simulink model "TRN_V3"  (R2022a)
settings: Solver=FixedStepAuto  StartTime=0.0  StopTime=300  FixedStep=0.04  RelTol=1e-3
PreLoadFcn:
  | load('BusStructureTRNsensor.mat')
InitFcn:
  | %load TRNDataBusPILS.mat
  | %addpath(genpath(cd))
  | 
  | % Add DataBus Path
  | addpath(',,/');
  | addpath('../MAP/');
  | addpath('../MAP/MAP_DB');
  | addpath('../MAP/DVOF');
  | addpath(genpath(cd));
  | load('BusStructureTRN.mat');
  | load('BusStructureDatapump.mat');
undefined symbols (not defined in the file or in its folder): Altitude_INS, INSDataNotValid, Latitude_INS, Longitude_INS, RALTValid, TRN, TRNlib
libraries: simulink_extras x38, aerolibconvert2 x20, dspstat3 x3, sharedtransform x2
(part 3 of 3)

== stateflow chart TRN_V3/TRN/TRNSchedulerDTNS1 ==
  state Operation_In_Flight
    state Check_On_Terrain_Map [parallel]
      en, du:  Out_TRNOutput.AircraftOffTerrainMap = CheckOffTerrainMap(In_TRNInput.Latitude_INS, In_TRNInput.Longitude_INS);
      settings: executionOrder=1
    state Terrain_Referenced_Navigation [parallel]
      settings: executionOrder=2
      state On_Terrain_Map
        state AcquisitionCSU
          state Batch_On
            state CollectProfile [parallel]
              en, du: [Out_TRNDatapump.MAD, Out_TRNDatapump.profileCnt, posUpdate, Out_TRNDatapump.residual] =...
              AcquisitionCSU(In_TRNInput,In_TRNDatapump)
              settings: executionOrder=1
            state CorrelationAnalysis [parallel]
              settings: executionOrder=2
              state BatchUpdate_On
                en, du: Out_TRNOutput.TRNEstOfINSLatitudeErr = -posUpdate(1) * 180/pi;
                Out_TRNOutput.TRNEstOfINSLongitudeErr = -posUpdate(2) * 180/pi;
                Out_TRNDatapump.profileCnt = 0;
                Out_TRNOutput.NavigationMode = false;
                Out_TRNOutput.AircraftPositionCorrectionValid = true;
                Out_Pmatrix = InitPmatrix();
              state BatchUpdate_Off
                en, du: Out_TRNOutput.TRNEstOfINSLatitudeErr = 0.0;
                Out_TRNOutput.TRNEstOfINSLongitudeErr = 0.0;
                Out_TRNOutput.NavigationMode = true;
                Out_TRNOutput.AircraftPositionCorrectionValid = false;
                Out_Pmatrix = InitPmatrix();
              (default) -> (junction 198)
              (junction 198) -> BatchUpdate_On [order 1] : [(Out_TRNDatapump.MAD <= 50&&...
                  | Out_TRNDatapump.profileCnt >= 20) || ...
                  |  (In_TRNInput.GPSDataNotValid == 0 && ...
                  | Out_TRNDatapump.MAD <= 50&&...
                  | Out_TRNDatapump.profileCnt >= 5)]
              (junction 198) -> BatchUpdate_Off [order 2]
          state Batch_Idle
            entry: Out_TRNOutput.TRNEstOfINSLatitudeErr = 0.0;
            Out_TRNOutput.TRNEstOfINSLongitudeErr = 0.0;
            Out_TRNOutput.NavigationMode = true;
            Out_TRNOutput.AircraftPositionCorrectionValid = false;
          (default) -> Batch_On
          Batch_Idle -> Batch_On : after(24, tick)
          Batch_On -> Batch_Idle : after(1, tick)
        state TrackingCSU
          state ContinuousUpdate [parallel]
            en,du:  [xu,Pmatrix,residual,latINSErrTRN,lonINSErrTRN, ...
            altINSErrTRN,hUncertainty,vUncertainty, Out_TRNDatapump.TimeTag_Prev, Out_TRNDatapump.Result_Prev] = ...
            TrackingCSU(In_TRNInput,In_Pmatrix,Qmatrix,Rmatrix, In_TRNDatapump);
            [continuousValid, Out_TRNOutput.NavigationMode]...
            = CheckValidity( hUncertainty, In_TRNInput.INSDataNotValid);
            settings: executionOrder=1
          state ValidityCheck [parallel]
            settings: executionOrder=2
            state ContinuousValid
              en, du:
              Out_TRNOutput.TRNEstOfINSLatitudeErr = latINSErrTRN * 180/pi;
              Out_TRNOutput.TRNEstOfINSLongitudeErr = lonINSErrTRN * 180/pi;
              Out_TRNOutput.TRNEstOfINSAltitudeErr = altINSErrTRN;
              Out_TRNOutput.AircraftPositionCorrectionValid = true;
            state ContinuousInValid
              en, du:
              Out_TRNOutput.TRNEstOfINSLatitudeErr = 0.0;
              Out_TRNOutput.TRNEstOfINSLongitudeErr = 0.0;
              Out_TRNOutput.TRNEstOfINSAltitudeErr = 0.0;
              Out_TRNOutput.AircraftPositionCorrectionValid = false;
            (default) -> ContinuousValid
            ContinuousValid -> ContinuousInValid : [continuousValid == false]
            ContinuousInValid -> ContinuousValid : [continuousValid == true]
          state UpdateContinuousParam [parallel]
            en, du:
            Out_TRNOutput.TRNHorUncertainty = hUncertainty * 6378000 * 25;
            Out_TRNOutput.TRNVerticalUncertainty = vUncertainty * 25;
            Out_TRNDatapump.xu = xu;
            Out_TRNDatapump.residual = residual;
            Out_Pmatrix = Pmatrix;
            %Out_TRNOutput.TRN_valid = TRN_valid;
            settings: executionOrder=3
        (default) -> AcquisitionCSU
        TrackingCSU -> AcquisitionCSU : [In_TRNOutput.NavigationMode == true]
        AcquisitionCSU -> TrackingCSU : [In_TRNOutput.NavigationMode == false]
      state Of_fTerrain_Map
      (default) -> On_Terrain_Map
      On_Terrain_Map -> Of_fTerrain_Map : [Out_TRNOutput.AircraftOffTerrainMap == true]
      Of_fTerrain_Map -> On_Terrain_Map : [Out_TRNOutput.AircraftOffTerrainMap == false]
  state Flight_Idle
    en, du:
    Out_TRNOutput.AircraftOffTerrainMap = CheckOffTerrainMap(In_TRNInput.Latitude_INS, In_TRNInput.Longitude_INS);
    Out_TRNOutput.TRN_valid = true;
    Out_TRNOutput.TRNEstOfINSLatitudeErr = 0.0;
    Out_TRNOutput.TRNEstOfINSLongitudeErr = 0.0;
    Out_TRNOutput.TRNEstOfINSAltitudeErr = 0.0;
    Out_TRNOutput.NavigationMode = false;
    Out_TRNOutput.AircraftPositionCorrectionValid = false;
  state [xu,Out_Pmatrix,residual,latINSErrTRN,lonINSErrTRN,altINSErrTRN,hUncertainty,vUncertainty,TimeTag_Prev,Result_Prev] = TrackingCSU(In_TRNInput,In_Pmatrix,Qmatrix,Rmatrix,In_TRNDatapump) [function]
  state [MAD,profileCnt,posUpdate,residual] = AcquisitionCSU(In_TRNInput,In_TRNDatapump) [function]
  (default) -> Operation_In_Flight
  Operation_In_Flight -> Flight_Idle : [In_TRNInput.WeightOnWheels == 1]
  Flight_Idle -> Operation_In_Flight : [In_TRNInput.WeightOnWheels == 0]
  data: In_TRNInput function_input Bus: TRNInput size=1 =0; In_Pmatrix function_input double size=[15 15]; Qmatrix function_input double size=[6 6]; Rmatrix function_input double size=1; xu function_output; Out_Pmatrix function_output; residual function_output; latINSErrTRN function_output; lonINSErrTRN function_output; altINSErrTRN function_output; hUncertainty function_output; vUncertainty function_output; In_TRNDatapump function_input Bus: TRNDatapump size=1; TimeTag_Prev function_output; Result_Prev function_output; In_TRNInput function_input Bus: TRNInput size=1 =0; In_TRNDatapump function_input Bus: TRNDatapump size=1 =0; MAD function_output; profileCnt function_output; posUpdate function_output; residual function_output; hUncertaintyTRN function_input; INSDataNotValid function_input; valid function_output; navigationMode function_output; Pmat function_output double size=[15 15]; lat function_input; lon function_input; AircraftOffTerrainMap function_output; In_TRNInput input Bus: TRNInput; In_TRNOutput input Bus: TRNOutput; In_TRNDatapump input Bus: TRNDatapump; In_Pmatrix input double size=[15 15]; Out_TRNOutput output Bus: TRNOutput; Out_TRNDatapump output Bus: TRNDatapump; Qmatrix input double size=[6 6]; Rmatrix input double size=1; vUncertainty local double; lonINSErrTRN local double; latINSErrTRN local double; hUncertainty local double; altINSErrTRN local double; posUpdate local double; continuousValid local boolean; residual local double; xu local double size=15; Pmatrix local double size=[15 15]; Out_Pmatrix output double size=[15 15]
  function [valid, navigationMode] = CheckValidity(hUncertaintyTRN, INSDataNotValid):
    | % function [valid, navigationMode] = CheckValidity(hUncertaintyTRN, vUncertaintyTRN, residualTRN)
    | 
    | % persistent invalidCnt
    | % if(isempty(invalidCnt))
    | %     invalidCnt = 0;
    | % end
    | % 
    | % weightedResidual = abs(residualTRN)/vUncertaintyTRN;
    | % 
    | % if(vUncertainty > 1 && weightedResidual > 35)
    | %     valid = false;
    | %     invalidCnt = invalidCnt + 1;
    | % else
    | %     valid = true;
    | %     invalidCnt = 0;
    | % end
    | % 
    | % if (invalidCnt >= 50)
    | %     navigationMode = true;
    | % else
    | %     navigationMode = false;
    | % end
    | % 
    | % end
    | 
    | function [valid, navigationMode] = CheckValidity(hUncertaintyTRN, INSDataNotValid)
    | 
    | persistent invalidCnt
    | if(isempty(invalidCnt))
    |     invalidCnt = 0;
    | end
    | 
    | if(hUncertaintyTRN > (256 * 6378000 * 25)) || INSDataNotValid == 1
    | % if(hUncertaintyTRN > (256))
    |     valid = false;
    |     invalidCnt = invalidCnt + 1;
    | else
    |     valid = true;
    |     invalidCnt = 0;
    | end
    | 
    | if (invalidCnt >= 50) || INSDataNotValid == 1
    |     navigationMode = true;        % Acq CSU
    | else
    |     navigationMode = false;       % Track CSU
    | end
    | 
    | end
  function Pmat = InitPmatrix:
    | function Pmat = InitPmatrix()
    | 
    | R0      = 6378000;
    | 
    | attBias = [0 0 0];
    | velBias = [0 0 0];
    | posBias = [10 10 13.3] .* [1/R0 1/R0 1];
    | gyroBias = [0.4848e-6 0.4848e-6 0.4848e-6];
    | accBias = [2.9430e-4 2.9430e-4 2.9430e-4];
    | 
    | % Pmat = diag(0.*[attBias velBias posBias gyroBias accBias].^2);
    | Pmat = diag([attBias velBias posBias gyroBias accBias].^2);
    | 
    | end
  function AircraftOffTerrainMap = CheckOffTerrainMap(lat, lon):
    | function AircraftOffTerrainMap = CheckOffTerrainMap(lat, lon)
    | 
    | AircraftTerrainMap = 0;
    | AircraftTerrainMap = coder.ceval('IsScanBoundary', lat, lon);     % InBoundary 1, NotBoundary 0
    | 
    | if(AircraftTerrainMap == 0)     % InBoundary 1, NotBoundary 0
    |     AircraftOffTerrainMap = true;
    | else
    |     AircraftOffTerrainMap = false;
    | end
    | 
    | end

== matlab function TRN_V3/TRN/TRNSchedulerDTNS1/AcquisitionCSU/AcquisitionCSU/CorrelationAnalysis function ==
  data: batchProfile input; posUpdate output; profileCnt input; MAD output; resolution input; gridSize input; residual output; batchProfile output; lonTemp output; latTemp output; hDEM output; sum output
function [posUpdate, MAD, residual, batchProfile, lonTemp,latTemp,hDEM, sum] = CorrelationAnalysis(batchProfile, profileCnt, resolution, gridSize)
r2d = 180/pi;

posUpdate   = zeros(2,1);
MAD         = single(0);
sum         = 0;
latTemp     = 0;
lonTemp     = 0;
hDEM        = 0;
bestIdx     = [-999 -999];

gridRes  = 0.1;
MADTemp = 9999*ones(1,8000);

for i = -gridSize : gridSize
    for j = -gridSize : gridSize
        
        latTemp = batchProfile(((profileCnt-1)*(3+(gridSize+gridSize+1)*(gridSize+gridSize+1))) + 2) + i*gridRes*resolution;
        lonTemp = batchProfile(((profileCnt-1)*(3+(gridSize+gridSize+1)*(gridSize+gridSize+1))) + 3) + j*gridRes*resolution;
        hDEM    = coder.ceval('GetElevation', latTemp*r2d, lonTemp*r2d);

        batchProfile(((profileCnt-1)*(3+(gridSize+gridSize+1)*(gridSize+gridSize+1))) + 3 + ((i + gridSize) * (gridSize+gridSize+1)) + (j + gridSize + 1)) = abs(batchProfile(((profileCnt-1)*(3+(gridSize+gridSize+1)*(gridSize+gridSize+1))) + 1) - hDEM );   
    end
end

for i = 1 : (gridSize+gridSize+1) * (gridSize+gridSize+1)
    sum = 0;
    for j = 1 : profileCnt
        sum = sum + batchProfile(((j-1)*(3+(gridSize+gridSize+1)*(gridSize+gridSize+1))) + (i+3));
    end
    
    MADTemp(1,i) = sum/single(profileCnt);
    
end

[minMAD, minIdx] = min(MADTemp);
MAD = single(minMAD);
bestIdx(1) = floor(minIdx/(gridSize+gridSize+1));
bestIdx(2) = minIdx - (bestIdx(1) * (gridSize+gridSize+1));

if bestIdx(2) == 0
    bestIdx(1) = bestIdx(1) - 1;
    bestIdx(2) = (gridSize+gridSize);
end
%
bestIdx(1) = bestIdx(1) - gridSize;
bestIdx(2) = bestIdx(2) - gridSize - 1;
posUpdate(1) = bestIdx(1)*gridRes*resolution;
posUpdate(2) = bestIdx(2)*gridRes*resolution;

residual = double(MAD);

end

== matlab function TRN_V3/TRN/TRNSchedulerDTNS1/TrackingCSU/TrackingCSU1/EKFupdate/MATLAB Function ==
  data: u input; y1 output; y2 output; y3 output
function [y1,y2,y3] = fcn(u)
    y = (u);
    yy = [y(7), y(8), y(9)];
    utm_lat2m_deg = 110961.7060516;   
    utm_lon2m_deg = 89476.51124;

    y1 = rad2deg(yy(1))*utm_lat2m_deg;
    y2 = rad2deg(yy(2))*utm_lon2m_deg;
    y3 = yy(3);

end

== matlab function TRN_V3/TRN/TRNSchedulerDTNS1/AcquisitionCSU/AcquisitionCSU/StoreProfile function ==
  data: batchProfile input; batchProfile output; profileCnt input; latINS input; lonINS input; altINS input; RALT input; profileCnt output; gridSize output; latGPS input; lonGPS input; altGPS input; flagGPS input; flagINS input
function [batchProfile, profileCnt, gridSize] = StoreProfile(batchProfile, profileCnt, latINS, lonINS, altINS, RALT, latGPS, lonGPS, altGPS, flagGPS, flagINS)

gridSize = 20;

if(profileCnt >= 20)
      
    profileCnt = uint32(19);
    
    for i = 0:profileCnt-1
   
        for j = 1 : (3 + (gridSize + gridSize + 1) * (gridSize + gridSize + 1))
            batchProfile(i * (3 + (gridSize + gridSize + 1) * (gridSize + gridSize + 1)) + j) = batchProfile((i+1) * (3 + (gridSize + gridSize + 1) * (gridSize + gridSize + 1)) + j);
        end
    end
            
end

if flagGPS == 1
    batchProfile((profileCnt*(3+((gridSize + gridSize + 1) * (gridSize + gridSize + 1)))) + 1) = altINS - RALT;
    batchProfile((profileCnt*(3+((gridSize + gridSize + 1) * (gridSize + gridSize + 1)))) + 2) = latINS;
    batchProfile((profileCnt*(3+((gridSize + gridSize + 1) * (gridSize + gridSize + 1)))) + 3) = lonINS;
elseif flagGPS == 0
    batchProfile((profileCnt*(3+((gridSize + gridSize + 1) * (gridSize + gridSize + 1)))) + 1) = altGPS - RALT;
    batchProfile((profileCnt*(3+((gridSize + gridSize + 1) * (gridSize + gridSize + 1)))) + 2) = latGPS;
    batchProfile((profileCnt*(3+((gridSize + gridSize + 1) * (gridSize + gridSize + 1)))) + 3) = lonGPS;
end

if flagINS == 0
    profileCnt = profileCnt + 1;
elseif flagINS == 1
    profileCnt = uint32(0);
end

end

== matlab function TRN_V3/TRN/TRNSchedulerDTNS1/TrackingCSU/TrackingCSU1/Earth_radius ==
  data: M output; N output; in_psi input
function [M, N] = Earth_radius(in_psi)

    a   = 6378137;          % Earth's equatorial radius
    b   = 6356752.314245;   % Earth's polar radius
    psi = in_psi;           % psi(latitude_GPS)
    M   = ((a*b)^2) / ( ( (a*cos(psi))^2 + (b*sin(psi))^2 )^(3/2) );    % radius  of  curvature  in  meridian
    N   = (a^2) / ( ( (a*cos(psi))^2 + (b*sin(psi))^2 )^(1/2) );        % radius  of  curvature  in  prime  vertical

end

== matlab function TRN_V3/TRN/TRNSchedulerDTNS1/TrackingCSU/TrackingCSU1/INS_Update_1553falt ==
  data: latINS input; latINS output; lonINS input; altINS input; velN input; velE input; velD input; TimeTag input; lonINS output; altINS output; dt input
function [latINS, lonINS, altINS] = fcn(latINS, lonINS, altINS, velN, velE, velD, TimeTag, dt)

R0 = 6378000;

if TimeTag(5) == 1
    latINS = latINS + (velN * dt) * 1/(R0+altINS);
    lonINS = lonINS + (velE * dt) * 1/(R0+altINS);
    altINS = altINS + (velD * dt) * 1/(R0+altINS);
end

== matlab function TRN_V3/TRN/RALTValidCheck/MATLAB Function6 ==
  data: residual input; sigma_3 input; RALT_valid output; count output; count input
function [RALT_valid, count] = RALTValidCheck(residual, sigma_3, count)

if abs(residual) >= sigma_3
    count = count + 1;
else
    count = 0;
end

if count > 7
    RALT_valid = boolean(false);
else
    RALT_valid = boolean(true);
end

== matlab function TRN_V3/TRN/INS//GPSFilter/MATLAB Function ==
  data: u input; yy output
function yy = fcn(u)
    y = diag(u);
    yy = [y(1), y(2), y(3)./(6378000)];

    yy = yy.*(6378000*25);

end

== matlab function TRN_V3/TRN/Multiple Model Adaptive Estimation ==
  data: WoW input; GPSDataNotValid input; TRN_INSEstErr input; out_Corr_Lat output; TRN_Pmat_Lat input; TRN_Pmat_Lon input; TRN_Pmat_Alt input; LCI_INSEstErr input; LCI_Pmat_Lat input; LCI_Pmat_Lon input; LCI_Pmat_Alt input; out_Corr_Lon output; out_Corr_Alt output; Weight output
function [out_Corr_Lat,out_Corr_Lon,out_Corr_Alt,Weight] = MMAE(WoW, GPSDataNotValid,TRN_INSEstErr,TRN_Pmat_Lat,TRN_Pmat_Lon,TRN_Pmat_Alt,LCI_INSEstErr,LCI_Pmat_Lat,LCI_Pmat_Lon,LCI_Pmat_Alt)

Weight_Lat   = TRN_Pmat_Lat/(LCI_Pmat_Lat+TRN_Pmat_Lat);
Weight_Lon   = TRN_Pmat_Lon/(LCI_Pmat_Lon+TRN_Pmat_Lon);
Weight_Alt   = TRN_Pmat_Alt/(LCI_Pmat_Alt+TRN_Pmat_Alt);

if GPSDataNotValid == 0 && WoW == 0     % TRN+INS/GPS
    out_Corr_Lat = (1-Weight_Lat)*TRN_INSEstErr(1) + Weight_Lat*LCI_INSEstErr(1);
    out_Corr_Lon = (1-Weight_Lon)*TRN_INSEstErr(2) + Weight_Lon*LCI_INSEstErr(2);
    out_Corr_Alt = (1-Weight_Alt)*TRN_INSEstErr(3) + Weight_Alt*LCI_INSEstErr(3);
else                                    % TRN
    out_Corr_Lat = TRN_INSEstErr(1);
    out_Corr_Lon = TRN_INSEstErr(2);
    out_Corr_Alt = TRN_INSEstErr(3);
end

Weight = [Weight_Lat Weight_Lon Weight_Alt];

== matlab function TRN_V3/TRN/TRNSchedulerDTNS1/TrackingCSU/TrackingCSU1/MATLAB Function1 ==
  data: Lat_GPS input; Lon_GPS input; Alt_GPS input; Lat output; Lat_INS input; Lon_INS input; Alt_INS input; GPSvalid input; Lon output; Alt output
function [Lat,Lon,Alt] = fcn(Lat_GPS,Lon_GPS,Alt_GPS,Lat_INS,Lon_INS,Alt_INS,GPSvalid)

if GPSvalid == 0
    Lat = Lat_GPS;
    Lon = Lon_GPS;
    Alt = Alt_GPS;
else
    Lat = Lat_INS;
    Lon = Lon_INS;
    Alt = Alt_INS;
end

== matlab function TRN_V3/TRN/TRNSchedulerDTNS1/TrackingCSU/TrackingCSU1/MATLAB Function2 ==
  data: TimeTag_Prev input; TimeTag_Prev output; GPSTimeTag input; INSTimeTag input; RALTTimeTag input
function TimeTag_Prev   = fcn(TimeTag_Prev,GPSTimeTag,INSTimeTag,RALTTimeTag)


TimeTag_Prev(4) = 0;
TimeTag_Prev(5) = 0;
TimeTag_Prev(6) = 0;

if TimeTag_Prev(1) == GPSTimeTag
    TimeTag_Prev(4) = 1;
end

if TimeTag_Prev(2) == INSTimeTag
    TimeTag_Prev(5) = 1;
end

if TimeTag_Prev(3) == RALTTimeTag
    TimeTag_Prev(6) = 1;
end

TimeTag_Prev(1) = GPSTimeTag;
TimeTag_Prev(2) = INSTimeTag;
TimeTag_Prev(3) = RALTTimeTag;

== matlab function TRN_V3/TRN/INS//GPSFilter/Fupdate Function ==
  data: velN input; Fmatrix output; velE input; velD input; lat input; alt input; accN input; accE input; accD input; OM input; M input; N input
% ---------------------------------------------------------------------- %
%                   F matrix update function
%
%   INPUT:
%       velN: North Velocity                                [m/s]
%       velE: East Velocity                                 [m/s]
%       velD: Down Velocity                                 [m/s]
%       lat: Latitude                                       [rad]
%       alt: Altitude                                       [m]
%       accN: North acceleration                            [m/ss]
%       accE: East acceleration                             [m/ss]
%       accD: Down acceleration                             [m/ss]
%       OM: Magnitude of the rotation rate of the Earth     [rad/s]
%       DCMbn: Rotational matrix(body frame to navigation frame)
%       M: radius  of  curvature  in  meridian
%       N: radius  of  curvature  in  prime  vertical      
%
%   OUTPUT:
%       Fmatrix: System matrix of Kalman Filter
%
% ---------------------------------------------------------------------- %
function Fmatrix = Fupdate(velN, velE, velD, lat, alt, accN, accE, accD, OM, M, N)

    e11 = 0;
    e12 = -((OM * sin(lat)) + (velE/(N+alt) * tan(lat)));
    e13 = velN/(M+alt);
    e21 = ((OM * sin(lat)) + (velE/(N+alt) * tan(lat)));
    e22 = 0;
    e23 = ((OM * cos(lat)) + (velE/(N+alt)));
    e31 = -velN/(M+alt);
    e32 = -(OM * cos(lat)) - (velE/(N+alt));
    e33 = 0;
    Fee = [e11 e12 e13; e21 e22 e23; e31 e32 e33;];
    
    e11 = 0;
    e12 = 1/((N+alt));
    e13 = 0;
    e21 = -1/((M+alt));
    e22 = 0 ;
    e23 = 0 ;
    e31 = 0 ;
    e32 = -tan(lat)/(N+alt) ;
    e33 = 0 ;
    Fev = [e11 e12 e13; e21 e22 e23; e31 e32 e33;];
    
    e11 = -OM * sin(lat);
    e12 = 0;
    e13 = -velE/(((N+alt))^2);
    e21 = 0 ;
    e22 = 0 ;
    e23 = velN/(((M+alt))^2);
    e31 =  -(OM*cos(lat)) - (velE/(((N+alt))*(cos(lat))^2));
    e32 = 0 ;
    e33 = (velE * tan(lat)) / ((N+alt)^2) ;
    Fer = [e11 e12 e13; e21 e22 e23; e31 e32 e33;];
    
    e11 = 0 ;
    e12 = -accD ;
    e13 = accE ;
    e21 = accD ;
    e22 = 0 ;
    e23 = -accN ;
    e31 = -accE ;
    e32 = accN ;
    e33 = 0 ;
    Fve = [e11 e12 e13; e21 e22 e23; e31 e32 e33;];
    
    e11 = velD/((M+alt));
    e12 = -2*((OM * sin(lat)) + ((velE/((N+alt))) * tan (lat))) ;
    e13 = velN/(M+alt) ;
    e21 = (2*OM * sin(lat)) + ( (velE/((N+alt))) * tan(lat) );
    e22 = (1/((N+alt))) * ((velN * tan(lat)) + velD) ;
    e23 = 2*OM * cos(lat) + (velE/((N+alt)));
    e31 = (-2*velN)/((M+alt));
    e32 = -2*(OM * cos(lat) +  (velE/((N+alt)))) ;
    e33 = 0;
    Fvv = [e11 e12 e13; e21 e22 e23; e31 e32 e33;];
    
    e11 = -velE*( (2*OM * cos(lat)) + (velE/(((N+alt))*(cos(lat))^2)));
    e12 = 0 ;
    e13 = (((velE^2)*tan(lat))/((N+alt)^2)) - ((velN*velD)/((M+alt)^2)) ;
    e21 = 2*OM *((velN*cos(lat)) - (velD*sin(lat))) + ((velN*velE) / (((N+alt))*(cos(lat))^2)) ;
    e22 = 0 ;
    e23 = ((-velE*velD)/((N+alt)^2))-((velN*velE*tan(lat))/((N+alt)^2));
    e31 = 2 * OM * velE * sin(lat);
    e32 = 0;
    e33 =  (((velE^2)/((N+alt)^2)) + ((velN^2)/((M+alt)^2)));
    Fvr = [e11 e12 e13; e21 e22 e23; e31 e32 e33;];
    
    Fre = zeros(3);
    
    e11 = 1/((M+alt));
    e12 = 0;
    e13 = 0;
    e21 = 0;
    e22 = 1/(((N+alt))*cos(lat));
    e23 = 0;
    e31 = 0;
    e32 = 0;
    e33 = -1;
    Frv = [e11 e12 e13; e21 e22 e23; e31 e32 e33;];
    
    e11 = 0;
    e12 = 0;
    e13 = -velN/(((M+alt))^2);
    e21 = (velE*tan(lat))/(((N+alt))*cos(lat));
    e22 = 0;
    e23 = -velE/((((N+alt))^2)*cos(lat));
    e31 = 0;
    e32 = 0;
    e33 = 0;
    Frr = [e11 e12 e13; e21 e22 e23; e31 e32 e33;];
              
    Fmatrix =  [Frr    Frv    Fre      ;
                Fvr    Fvv    Fve      ;
                Fer    Fev    Fee      ];
        
end

== matlab function TRN_V3/TRN/INS//GPSFilter/Gupdate Function ==
  data: DCMbn input; Gmatrix output
% ---------------------------------------------------------------------- %
%                   G matrix update function
%
%   INPUT:
%       DCMbn: Rotational matrix(body frame to navigation frame)
%
%   OUTPUT:
%       Gmatrix: Input matrix of Kalman Filter
%
% ---------------------------------------------------------------------- %
function Gmatrix = Gupdate(DCMbn)

Z  = zeros(3);

Gmatrix =  [    Z       Z;
              DCMbn     Z;
                Z    -DCMbn;];

end

== matlab function TRN_V3/TRN/INS//GPSFilter/MesurementUpdate Function ==
  data: Lat_GPS input; Hmatrix output; Lon_GPS input; z output; alt_GPS input; velN_GPS input; velE_GPS input; velD_GPS input; Lat_INS input; Lon_INS input; alt_INS input; velN_INS input; velE_INS input; velD_INS input; M input; N input; psi input
function [Hmatrix, z] = MeasurementUpdate(Lat_GPS, Lon_GPS, alt_GPS, velN_GPS, velE_GPS, velD_GPS, ...
                                          Lat_INS, Lon_INS, alt_INS, velN_INS, velE_INS, velD_INS, ...
                                          M, N, psi)

alt = alt_INS;

Z   = zeros(3);
I   = eye(3);
H   = [(M+alt)        0             0;
         0     (N+alt)*cos(psi)     0;
         0            0             1;];

% H matrix
Hmatrix = [ H Z Z
            Z I Z]; 

z = [(M+alt)*(Lat_INS-Lat_GPS); 
    (N+alt)*cos(psi)*(Lon_INS-Lon_GPS);
     alt_INS - alt_GPS;
    velN_INS - velN_GPS;
    velE_INS - velE_GPS;
    velD_INS - velD_GPS;];


end

== matlab function TRN_V3/TRN/INS//GPSFilter/MesurementUpdate Function1 ==
  data: M output; N output; psi output; in_psi input
function [M, N, psi] = Earth_radius(in_psi)

    a   = 6378137;          % Earth's equatorial radius
    b   = 6356752.314245;   % Earth's polar radius
    psi = in_psi;           % psi(latitude_GPS)
    M   = ((a*b)^2) / ( ( (a*cos(psi))^2 + (b*sin(psi))^2 )^(3/2) );    % radius  of  curvature  in  meridian
    N   = (a^2) / ( ( (a*cos(psi))^2 + (b*sin(psi))^2 )^(1/2) );        % radius  of  curvature  in  prime  vertical

end

== matlab function TRN_V3/TRN/INS//GPSFilter/MesurementUpdate Function2 ==
  data: Lat_LCI output; Lat_INS input; Lon_INS input; alt_INS input; Lon_LCI output; alt_LCI output; Lat_LCI input; Lon_LCI input; alt_LCI input
function [Lat_LCI, Lon_LCI, alt_LCI] = MeasurementUpdate(Lat_INS, Lon_INS, alt_INS, ...
                                                                      Lat_LCI, Lon_LCI, alt_LCI)
    Lat_LCI = Lat_INS  - Lat_LCI;
    Lon_LCI = Lon_INS  - Lon_LCI;
    alt_LCI = alt_INS  - alt_LCI;

end

== matlab function TRN_V3/TRN/INS//GPSFilter/Rupdate Function ==
  data: Lat_GPS input; Rmatrix output; Lon_GPS input; alt_GPS input; velN_GPS input; velE_GPS input; velD_GPS input
% ---------------------------------------------------------------------- %
%                   R matrix update function
% ---------------------------------------------------------------------- %
function Rmatrix = Rupdate(Lat_GPS, Lon_GPS, alt_GPS, velN_GPS, velE_GPS, velD_GPS)

%     Rmatrix = diag([ std(Lat_GPS)^2 std(Lon_GPS)^2 std(alt_GPS)^2 std(velN_GPS)^2 std(velE_GPS)^2 std(velD_GPS)^2 ]);
%     Rmatrix = diag([ (6.6/sqrt(25))^2 (6.6/sqrt(25))^2 (6.6/sqrt(25))^2 (6.6/sqrt(25))^2 (6.6/sqrt(25))^2 (6.6/sqrt(25))^2 ]);
    Rmatrix = diag([ (6.6/sqrt(25))^2 (6.6/sqrt(25))^2 (1/sqrt(25))^2 (0.5/sqrt(25))^2 (0.5/sqrt(25))^2 (0.5/sqrt(25))^2 ]);
%     Rmatrix = diag([ (6.6/sqrt(25))^2 (6.6/sqrt(25))^2 (6.6/sqrt(25))^2 (0.0)^2 (0.0)^2 (0.0)^2 ]);

end

== matlab function TRN_V3/TRN/TRNSchedulerDTNS1/TrackingCSU/TrackingCSU1/EKFupdate/EKFUpdate Function ==
  data: z input; xu output; xp output; P output; F input; H input; G input; P input; Q input; R input; dt input; residual output; latINSErrTRN output; lonINSErrTRN output; altINSErrTRN output; hUncertainty output; vUncertainty output; xu_prev input; TimeTag input
function [xu, xp, P, residual, latINSErrTRN, lonINSErrTRN, altINSErrTRN, ...
          hUncertainty, vUncertainty] = EKFUpdate(z, F, H, G, P, Q, R, dt, xu_prev, TimeTag)

x = zeros(15,1);
I = eye(max(size(F)));

A = I + (F*dt);
Q = (A*G * Q * G'*A') .* dt;

%-------------------------------------%
% Predicts states & covariance matrix
%-------------------------------------%
xp = A * x;
Pp = (A * P * A') + Q;

%---------------------%
% Updates Kalman gain
%---------------------%
K = (Pp * H')/(R + H * Pp * H');

%----------------%
% Updates states
%----------------%
xu = xp + K * (z - H*xp);
% residual = z - H*xp;
residual = z;

%---------------------------%
% Updates covariance matrix
%---------------------------%
P = (I - K*H) * Pp * (I - K*H)' + K*R*K';


latINSErrTRN = xu(7);
lonINSErrTRN = xu(8);
altINSErrTRN = xu(9);
hUncertainty = sqrt(abs(P(7,7) + P(8,8)));
vUncertainty = sqrt(abs(P(9,9)));
AGLErrTRN    = uint16(vUncertainty+ sqrt(R)*randn(1));

if TimeTag(6) == 1
    xu = xu_prev;
    latINSErrTRN = xu(7);
    lonINSErrTRN = xu(8);
    altINSErrTRN = xu(9);
end

end

== matlab function TRN_V3/TRN/TRNSchedulerDTNS1/TrackingCSU/TrackingCSU1/Measurement/Fupdate Function ==
  data: velN input; Fmatrix output; velE input; velD input; lat input; alt input; accN input; accE input; accD input; OM input; R0 input; DCMbn input; M input; N input
% ---------------------------------------------------------------------- %
%                   F matrix update function
%
%   INPUT:
%       velN: North Velocity                                [m/s]
%       velE: East Velocity                                 [m/s]
%       velD: Down Velocity                                 [m/s]
%       lat: Latitude                                       [rad]
%       alt: Altitude                                       [m]
%       accN: North acceleration                            [m/ss]
%       accE: East acceleration                             [m/ss]
%       accD: Down acceleration                             [m/ss]
%       OM: Magnitude of the rotation rate of the Earth     [rad/s]
%       R0: Radius of Earth                                 [m]
%       DCMbn: Rotational matrix(body frame to navigation frame)
%
%   OUTPUT:
%       Fmatrix: System matrix of Kalman Filter
%
% ---------------------------------------------------------------------- %
function Fmatrix = Fupdate(velN, velE, velD, lat, alt, accN, accE, accD, OM, R0, DCMbn, M, N)
    
        Z  = zeros(3);
    
        e11 = 0;
        e12 = -((OM * sin(lat)) + (velE/(N+alt) * tan(lat)));
        e13 = velN/(M+alt);
        e21 = ((OM * sin(lat)) + (velE/(N+alt) * tan(lat)));
        e22 = 0;
        e23 = ((OM * cos(lat)) + (velE/(N+alt)));
        e31 = -velN/(M+alt);
        e32 = -(OM * cos(lat)) - (velE/(N+alt));
        e33 = 0;
        Fee = [e11 e12 e13; e21 e22 e23; e31 e32 e33;];
    
        e11 = 0;
        e12 = 1/((N+alt));
        e13 = 0;
        e21 = -1/((M+alt));
        e22 = 0 ;
        e23 = 0 ;
        e31 = 0 ;
        e32 = -tan(lat)/(N+alt) ;
        e33 = 0 ;
        Fev = [e11 e12 e13; e21 e22 e23; e31 e32 e33;];
    
        e11 = -OM * sin(lat);
        e12 = 0;
        e13 = -velE/(((N+alt))^2);
        e21 = 0 ;
        e22 = 0 ;
        e23 = velN/(((M+alt))^2);
        e31 =  -(OM*cos(lat)) - (velE/(((N+alt))*(cos(lat))^2));
        e32 = 0 ;
        e33 = (velE * tan(lat)) / ((N+alt)^2) ;
        Fep = [e11 e12 e13; e21 e22 e23; e31 e32 e33;];
    
        e11 = 0 ;
        e12 = -accD ;
        e13 = accE ;
        e21 = accD ;
        e22 = 0 ;
        e23 = -accN ;
        e31 = -accE ;
        e32 = accN ;
        e33 = 0 ;
        Fve = [e11 e12 e13; e21 e22 e23; e31 e32 e33;];
    
        e11 = velD/((M+alt));
        e12 = -2*((OM * sin(lat)) + ((velE/((N+alt))) * tan (lat))) ;
        e13 = velN/(M+alt) ;
        e21 = (2*OM * sin(lat)) + ( (velE/((N+alt))) * tan(lat) );
        e22 = (1/((N+alt))) * ((velN * tan(lat)) + velD) ;
        e23 = 2*OM * cos(lat) + (velE/((N+alt)));
        e31 = (-2*velN)/((M+alt));
        e32 = -2*(OM * cos(lat) +  (velE/((N+alt)))) ;
        e33 = 0;
        Fvv = [e11 e12 e13; e21 e22 e23; e31 e32 e33;];
    
        e11 = -velE*( (2*OM * cos(lat)) + (velE/(((N+alt))*(cos(lat))^2)));
        e12 = 0 ;
        e13 = (((velE^2)*tan(lat))/((N+alt)^2)) - ((velN*velD)/((M+alt)^2)) ;
        e21 = 2*OM *((velN*cos(lat)) - (velD*sin(lat))) + ((velN*velE) / (((N+alt))*(cos(lat))^2)) ;
        e22 = 0 ;
        e23 = ((-velE*velD)/((N+alt)^2))-((velN*velE*tan(lat))/((N+alt)^2));
        e31 = 2 * OM * velE * sin(lat);
        e32 = 0;
        e33 =  (((velE^2)/((N+alt)^2)) + ((velN^2)/((M+alt)^2)));
        Fvp = [e11 e12 e13; e21 e22 e23; e31 e32 e33;];
    
        Fpe = zeros(3);
    
        e11 = 1/((M+alt));
        e12 = 0;
        e13 = 0;
        e21 = 0;
        e22 = 1/(((N+alt))*cos(lat));
        e23 = 0;
        e31 = 0;
        e32 = 0;
        e33 = -1;
        Fpv = [e11 e12 e13; e21 e22 e23; e31 e32 e33;];
    
        e11 = 0;
        e12 = 0;
        e13 = -velN/(((M+alt))^2);
        e21 = (velE*tan(lat))/(((N+alt))*cos(lat));
        e22 = 0;
        e23 = -velE/((((N+alt))^2)*cos(lat));
        e31 = 0;
        e32 = 0;
        e33 = 0;
        Fpp = [e11 e12 e13; e21 e22 e23; e31 e32 e33;];
    
    
        %     Fvv = zeros(3);
        %     Fvp = zeros(3);
        %     Fpp = zeros(3);
    
        Fmatrix =  [Fee    Fev    Fep      DCMbn          Z      ;
                    Fve    Fvv    Fvp        Z           DCMbn   ;
                    Fpe    Fpv    Fpp        Z            Z      ;
                    Z      Z      Z          Z            Z      ;
                    Z      Z      Z          Z            Z      ;];


end

== matlab function TRN_V3/TRN/TRNSchedulerDTNS1/TrackingCSU/TrackingCSU1/Measurement/Gupdate Function ==
  data: DCMbn input; Gmatrix output
% ---------------------------------------------------------------------- %
%                   G matrix update function
%
%   INPUT:
%       DCMbn: Rotational matrix(body frame to navigation frame)
%
%   OUTPUT:
%       Gmatrix: Input matrix of Kalman Filter
%
% ---------------------------------------------------------------------- %
function Gmatrix = Gupdate(DCMbn)

Z  = zeros(3);
I  = eye(3);

Gmatrix =  [ -DCMbn     Z;
                Z      DCMbn;
                Z       Z;
                Z       Z;
                Z       Z;];      

end

== matlab function TRN_V3/TRN/TRNSchedulerDTNS1/TrackingCSU/TrackingCSU1/Measurement/MATLAB Function1 ==
  data: RALTValid input; roll input; pitch input; z_out output; z_in input
function z_out = fcn(RALTValid, roll, pitch, z_in)

z_out = 0;

if RALTValid == true && abs(roll) < deg2rad(15) && abs(pitch) < deg2rad(15)
    z_out = z_in;

else
    z_out = 0;
end

== matlab function TRN_V3/TRN/TRNSchedulerDTNS1/TrackingCSU/TrackingCSU1/Measurement/MesurementUpdate Function ==
  data: Hmatrix output; lat input; lon input; alt input; RALT input; z output
% function [Hmatrix, z, hDEM] = MeasurementUpdate(resolution, lat, lon, alt, RALT)
function [Hmatrix, z] = MeasurementUpdate(lat, lon, alt, RALT)

%% DTRAN
%     P11 = 0;
%     P12 = 0;    
%     P21 = 0;    
%     P22 = 0;
%     
%     x = mod( (lon - leftLon)/resolution, 1 )*resolution;  y = mod( (lat - bottomLat)/resolution, 1)*resolution;
%     
%     leftLonIndex   =   floor( (lon - leftLon)/resolution );
%     lowerLatIndex  =   floor( (lat - bottomLat)/resolution );
%     
%     P11 = coder.ceval('GetElevationFromIndex', lowerLatIndex, leftLonIndex);
%     P12 = coder.ceval('GetElevationFromIndex', lowerLatIndex, leftLonIndex+1);
%     P21 = coder.ceval('GetElevationFromIndex', lowerLatIndex+1, leftLonIndex);
%     P22 = coder.ceval('GetElevationFromIndex', lowerLatIndex+1, leftLonIndex+1);
%     
%     if P11 < -12000 || P11 > 9000
%         P11 = 0;
%     end
%     if P12 < -12000 || P12 > 9000
%         P12 = 0;
%     end
%     if P21 < -12000 || P21 > 9000
%         P21 = 0;
%     end
%     if P22 < -12000 || P22 > 9000
%         P22 = 0;
%     end
%     
%     P_low    =   (resolution-x)/resolution * P11    +   (x/resolution) * P12;
%     P_high   =   (resolution-x)/resolution * P21    +   (x/resolution) * P22;
%     P_left   =   (resolution-y)/resolution * P11    +   (y/resolution) * P21;
%     P_right  =   (resolution-y)/resolution * P12    +   (y/resolution) * P22;
%     
%     hdot_lat    =   (P_high - P_low) / resolution;
%     hdot_lon    =   (P_right - P_left) / resolution;
%     
%     % H matrix
%     Hmatrix     =  [ zeros(1,6) -hdot_lat   -hdot_lon    1  zeros(1,6) ]; 
%     
%     hDEM = (resolution-y)/resolution * P_low  +   (y/resolution) * P_high;
%     
%     z = (alt - hDEM) - RALT;

%% DTNS
    P_low = 0.0;
    P_high = 0.0;    
    P_left = 0.0;    
    P_right = 0.0;
    hDEM = double(0.0);         
    resultDTED = uint32(1);
    resultDVOF = int32(1);

    resolution = 3 * 0.000277777777777777;

    lat = rad2deg(lat);
    lon = rad2deg(lon);
    
    resultDVOF = coder.ceval('UpdateObstList', lat, lon);
    resultDTED = coder.ceval('UpdateMapCache', lat, lon);
    
    P_low    =   coder.ceval('GetElevation', lat - resolution, lon);
    P_high   =   coder.ceval('GetElevation', lat + resolution, lon);
    P_left   =   coder.ceval('GetElevation', lat, lon - resolution);
    P_right  =   coder.ceval('GetElevation', lat, lon + resolution);
    
    hdot_lat    =   (P_high - P_low) / resolution;
    hdot_lon    =   (P_right - P_left) / resolution;
    
    % H matrix
    Hmatrix     =  [ zeros(1,6) -hdot_lat   -hdot_lon    1  zeros(1,6) ]; 
    
    hDEM = coder.ceval('GetElevation', lat, lon);
    
    z = (alt - hDEM) - RALT;

end

== matlab function TRN_V3/TRN/INS//GPSFilter/MATLAB Function1 ==
  data: GPSValid input; z_out output; z_in input; Lat_GPS input; Lat_GPS_temp input; Lon_GPS input; Lon_GPS_temp input
function z_out = fcn(GPSValid, z_in, Lat_GPS, Lat_GPS_temp, Lon_GPS, Lon_GPS_temp)

z_out = zeros(6,1);

if GPSValid == 0    % GPS valid
    if (abs(rad2deg(Lat_GPS - Lat_GPS_temp)) < 0.000000001) || (abs(rad2deg(Lon_GPS - Lon_GPS_temp)) < 0.000000001)    % Propagation  
        z_out = zeros(6,1);
    else                % Update
        z_out = z_in;
    end   
    
else
    z_out = zeros(6,1);
end

== matlab function TRN_V3/TRN/INS//GPSFilter/ConvertINSInput/MATLAB Function2 ==
  data: TimeTag_Prev input; TimeTag_Prev output; GPSTimeTag input; INSTimeTag input; RALTTimeTag input
function TimeTag_Prev   = fcn(TimeTag_Prev,GPSTimeTag,INSTimeTag,RALTTimeTag)


TimeTag_Prev(4) = 0;
TimeTag_Prev(5) = 0;
TimeTag_Prev(6) = 0;

if TimeTag_Prev(1) == GPSTimeTag
    TimeTag_Prev(4) = 1;
end

if TimeTag_Prev(2) == INSTimeTag
    TimeTag_Prev(5) = 1;
end

if TimeTag_Prev(3) == RALTTimeTag
    TimeTag_Prev(6) = 1;
end

TimeTag_Prev(1) = GPSTimeTag;
TimeTag_Prev(2) = INSTimeTag;
TimeTag_Prev(3) = RALTTimeTag;

== matlab function TRN_V3/TRN/TRNSchedulerDTNS1/TrackingCSU/TrackingCSU1/EKFupdate/MATLAB Function1 ==
  data: u input; y1 output; y2 output; y3 output
function [y1,y2,y3] = fcn(u)
    y = (u);
    yy = [y(7), y(8), y(9)];
    utm_lat2m_deg = 110961.7060516;   
    utm_lon2m_deg = 89476.51124;

    y1 = rad2deg(yy(1))*utm_lat2m_deg;
    y2 = rad2deg(yy(2))*utm_lon2m_deg;
    y3 = yy(3);

end
